simulink model "Practica1"  (R2015a)
settings: Solver=ode45  StartTime=0.0  StopTime=8.0  RelTol=1e-3
libraries: simulink x1
settings Model: Creator=redes  LastModifiedBy=redes

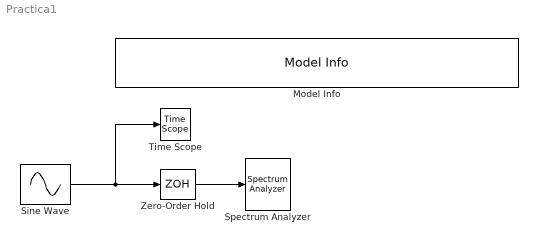
== system Practica1 ==
  Model Info : simulink/Model-Wide Utilities/Model Info  Frame=on  DisplayStringWithTags=Resolución práctica 1. Señales en el tiempo y frecuencia  HorizontalTextAlignment=Center  LeftAlignmentValue=0.5  SourceBlockDiagram=Practica1  TagMaxNumber=20
  Sine Wave : Sin  Amplitude=1.5  Frequency=2*pi*30  Phase=pi  SampleTime=0.0025
  Spectrum Analyzer : SpectrumAnalyzer
  Time Scope : TimeScope  DefaultConfigurationName=spbscopes.TimeScopeBlockCfg
  Zero-Order Hold : ZeroOrderHold  SampleTime=0.0025
  wires:
  Sine Wave/1 -> Zero-Order Hold/1, Time Scope/1
  Zero-Order Hold/1 -> Spectrum Analyzer/1
